simulink library "INT_InjCrv_PiI2AddCor"  (R2016b)
settings: Solver=VariableStepAuto  StartTime=0.0  StopTime=10.0  RelTol=1e-3
settings Model: Creator=zhoutinglin  LastModifiedBy=zhoutinglin

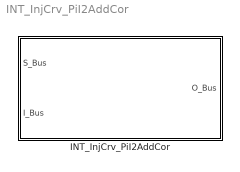
== system INT_InjCrv_PiI2AddCor ==
  INT_InjCrv_PiI2AddCor : Subsystem

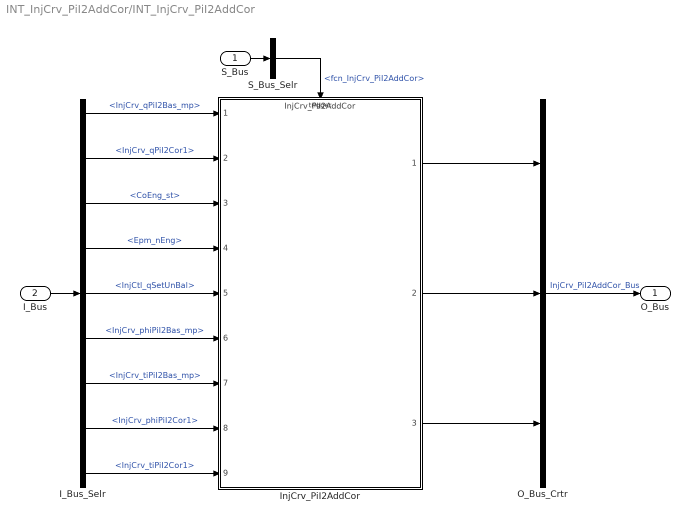
== system INT_InjCrv_PiI2AddCor/INT_InjCrv_PiI2AddCor ==
  S_Bus : Inport
  I_Bus : Inport  Port=2
  I_Bus_Selr : BusSelector  OutputSignals=InjCrv_qPiI2Bas_mp,InjCrv_qPiI2Cor1,CoEng_st,Epm_nEng,InjCtl_qSetUnBal,InjCrv_phiPiI2Bas_mp,InjCrv_tiPiI2Bas_mp,InjCrv_phiPiI2Cor1,InjCrv_tiPiI2Cor1
  InjCrv_PiI2AddCor : ModelReference  ModelNameDialog=InjCrv_PiI2AddCor  SimulationMode=Normal  ModelReferenceVersion=1.27  TriggerPortName=function  TriggerPortTriggerType=function-call  TriggerPortStatesWhenEnabling=held
  O_Bus_Crtr : BusCreator  Inputs=3
  S_Bus_Selr : BusSelector  OutputSignals=fcn_InjCrv_PiI2AddCor
  O_Bus : Outport
  wires:
  S_Bus_Selr/1 -> InjCrv_PiI2AddCor/Trigger  "<fcn_InjCrv_PiI2AddCor>"
  S_Bus/1 -> S_Bus_Selr/1
  I_Bus/1 -> I_Bus_Selr/1
  I_Bus_Selr/1 -> InjCrv_PiI2AddCor/1  "<InjCrv_qPiI2Bas_mp>"
  I_Bus_Selr/2 -> InjCrv_PiI2AddCor/2  "<InjCrv_qPiI2Cor1>"
  I_Bus_Selr/3 -> InjCrv_PiI2AddCor/3  "<CoEng_st>"
  I_Bus_Selr/4 -> InjCrv_PiI2AddCor/4  "<Epm_nEng>"
  I_Bus_Selr/5 -> InjCrv_PiI2AddCor/5  "<InjCtl_qSetUnBal>"
  I_Bus_Selr/6 -> InjCrv_PiI2AddCor/6  "<InjCrv_phiPiI2Bas_mp>"
  I_Bus_Selr/7 -> InjCrv_PiI2AddCor/7  "<InjCrv_tiPiI2Bas_mp>"
  I_Bus_Selr/8 -> InjCrv_PiI2AddCor/8  "<InjCrv_phiPiI2Cor1>"
  I_Bus_Selr/9 -> InjCrv_PiI2AddCor/9  "<InjCrv_tiPiI2Cor1>"
  O_Bus_Crtr/1 -> O_Bus/1  "InjCrv_PiI2AddCor_Bus"
  InjCrv_PiI2AddCor/1 -> O_Bus_Crtr/1
  InjCrv_PiI2AddCor/2 -> O_Bus_Crtr/2
  InjCrv_PiI2AddCor/3 -> O_Bus_Crtr/3
